simulink model "ultra"  (R2020b)
settings: Solver=FixedStepDiscrete  StartTime=0.0  StopTime=10.0  FixedStep=0.0005  RelTol=1e-3  EnableMultiTasking=on
undefined symbols (not defined in the file): acc_calmax1, acc_calmax2, acc_calmin1, acc_calmin2, akemancanshu, bre, bre_calmax, bre_calmin, ecucoder_acal, I_AN01_5K1, I_AN03_5V, I_AN04_5V, kd, ki, kp, leftmax, O_SW06_HS1A, rightmax, T_add, T_del, tiaoshi, zhiling
libraries: ec5744lib x215, canmsglib x75, simulink x10
(part 1 of 7)
settings Model: Creator=Tom liu  LastModifiedBy=Liu keliang
settings OptimizationCC: DefaultParameterBehavior=Inlined  UseDivisionForNetSlopeComputation=on  GainParamInheritBuiltInType=on  UseFloatMulNetSlope=on  InlineInvariantSignals=on  EnhancedBackFolding=on  ExpressionFolding=off  PassReuseOutputArgsAs=Individual arguments  RollThreshold=65  StateBitsets=on  DataBitsets=on  ZeroExternalMemoryAtStartup=off  ZeroInternalMemoryAtStartup=off  NoFixptDivByZeroProtection=on  EfficientFloat2IntCast=on  OptimizeBlockOrder=speed  DifferentSizesBufferReuse=on  EfficientTunableParamExpr=on
settings DebuggingCC: InheritedTsInSrcMsg=none  MultiTaskDSMMsg=none  ParameterTunabilityLossMsg=error
settings HardwareCC: ProdBitPerPointer=32  ProdBitPerSizeT=32  ProdBitPerPtrDiffT=32  ProdLargestAtomicInteger=Long  ProdLargestAtomicFloat=Double  ProdEndianess=BigEndian  ProdWordSize=32  ProdHWDeviceType=Freescale MPC5500  TargetBitPerPointer=64  TargetBitPerSizeT=64  TargetBitPerPtrDiffT=64  TargetLongLongMode=on  TargetIntDivRoundTo=Zero  TargetEndianess=LittleEndian  TargetWordSize=64  TargetHWDeviceType=MATLAB Host  ProdEqTarget=off
settings SFSimCC: MATLABDynamicMemAlloc=off  CustomCodeUndefinedFunction=UseInterfaceOnly
settings RTWCC: Description=Target for EC5744  SystemTargetFile=ec5744.tlc  MakeCommand=make_rtw optimized_fixed_point=1  GenerateMakefile=off  TemplateMakefile=ec5744_lcc.tmf  PostCodeGenCommand=ec5744_pst_s2(buildInfo)  GenerateReport=on  IncludeHyperlinkInReport=on  LaunchReport=on
settings CodeAppCC: ForceParamTrailComments=on  IgnoreCustomStorageClasses=off  OperatorAnnotations=on  SimulinkDataObjDesc=on  SFDataObjDesc=on  CustomSymbolStrGlobalVar=rt$N$M  CustomSymbolStrType=$N$M  CustomSymbolStrFcn=$N$M$F  CustomSymbolStrMacro=$N$M  InsertBlockDesc=on
settings STFCustomTargetCC: TargetLangStandard=C99 (ISO)  MultiwordLength=256  ModelReferenceCompliant=off  ConcurrentExecutionCompliant=off  IncludeMdlTerminateFcn=off  CombineOutputUpdateFcns=on  SuppressErrorStatus=on  ERTCustomFileBanners=on  SupportContinuousTime=off  SupportNonInlinedSFcns=off  RemoveResetFunc=on  MATLABClassNameForMDSCustomization=Simulink.SoftwareTarget.ERTCustomization  CPPClassGenCompliant=off  GRTInterface=off  SystemTargetFile=ec5744.tlc
settings ERTTargetCC: TargetLangStandard=C99 (ISO)  ModelReferenceCompliant=off  ParMdlRefBuildCompliant=off  CompOptLevelCompliant=off  ConcurrentExecutionCompliant=off  IncludeMdlTerminateFcn=off  SuppressErrorStatus=on  ModelStepFunctionPrototypeControlCompliant=off  CPPClassGenCompliant=off  UseToolchainInfoCompliant=off  GenerateASAP2=on  InlinedParameterPlacement=NonHierarchical  ERTSrcFileBannerTemplate=ec5744_code_template.cgt  ERTHdrFileBannerTemplate=ec5744_code_template.cgt  ERTDataSrcFileTemplate=ec5744_code_template.cgt  ERTDataHdrFileTemplate=ec5744_code_template.cgt  ERTCustomFileTemplate=ec5744_file_process.tlc

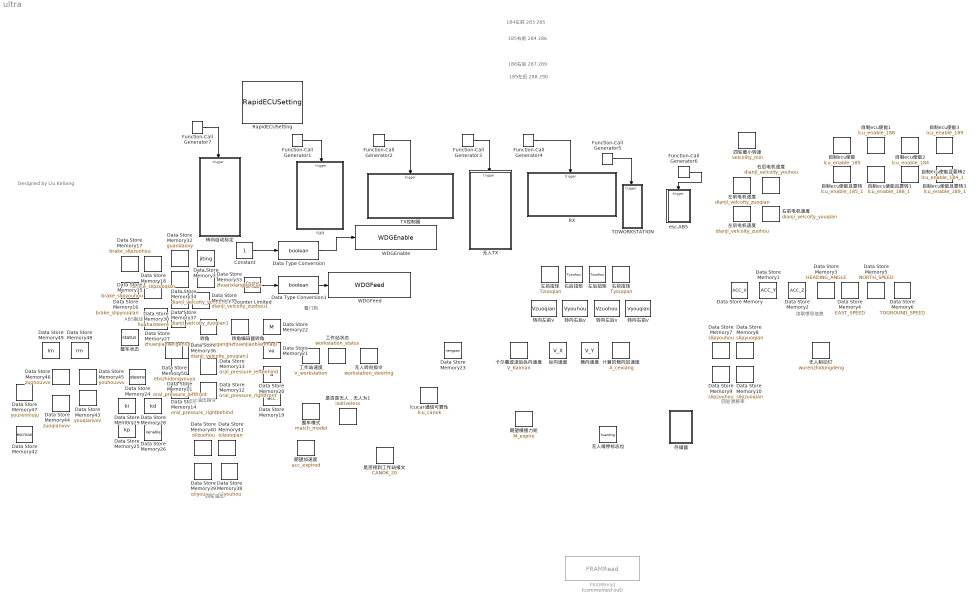
== system ultra ==
  note: Designed by Liu Keliang
  note: 四轮油压
  note: ABS制动
  note: esc油压指令
  note: 四轮滑移率
  note: 读取惯导信息
  note: 看门狗
  note: 189左后 288 290
  note: 188右后 287 289
  note: 185右前 284 286
  note: 184左前 283 285
  Constant : Constant
  Counter Limited : simulink/Sources/Counter Limited  uplimit=1  tsamp=0.01
  Data Store Memory : DataStoreMemory  DataStoreName=ACC_X  ReadBeforeWriteMsg=warning  WriteAfterWriteMsg=warning  WriteAfterReadMsg=warning  ShowAdditionalParam=off
  Data Store Memory1 : DataStoreMemory  DataStoreName=ACC_Y  ReadBeforeWriteMsg=warning  WriteAfterWriteMsg=warning  WriteAfterReadMsg=warning  ShowAdditionalParam=off
  Data Store Memory10 : DataStoreMemory  DataStoreName=slipzuoqian  ReadBeforeWriteMsg=warning  WriteAfterWriteMsg=warning  WriteAfterReadMsg=warning  ShowAdditionalParam=off
  Data Store Memory11 : DataStoreMemory  DataStoreName=oral_pressure_leftfront  ReadBeforeWriteMsg=warning  WriteAfterWriteMsg=warning  WriteAfterReadMsg=warning  ShowAdditionalParam=off
  Data Store Memory12 : DataStoreMemory  DataStoreName=oral_pressure_rightfront  ReadBeforeWriteMsg=warning  WriteAfterWriteMsg=warning  WriteAfterReadMsg=warning  ShowAdditionalParam=off
  Data Store Memory13 : DataStoreMemory  DataStoreName=oral_pressure_leftbehind  ReadBeforeWriteMsg=warning  WriteAfterWriteMsg=warning  WriteAfterReadMsg=warning  ShowAdditionalParam=off
  Data Store Memory14 : DataStoreMemory  DataStoreName=oral_pressure_rightbehind  ReadBeforeWriteMsg=warning  WriteAfterWriteMsg=warning  WriteAfterReadMsg=warning  ShowAdditionalParam=off
  Data Store Memory15 : DataStoreMemory  DataStoreName=brake_slipyouhou  ReadBeforeWriteMsg=warning  WriteAfterWriteMsg=warning  WriteAfterReadMsg=warning  ShowAdditionalParam=off
  Data Store Memory16 : DataStoreMemory  DataStoreName=brake_slipyouqian  ReadBeforeWriteMsg=warning  WriteAfterWriteMsg=warning  WriteAfterReadMsg=warning  ShowAdditionalParam=off
  Data Store Memory17 : DataStoreMemory  DataStoreName=brake_slipzuohou  ReadBeforeWriteMsg=warning  WriteAfterWriteMsg=warning  WriteAfterReadMsg=warning  ShowAdditionalParam=off
  Data Store Memory18 : DataStoreMemory  DataStoreName=brake_slipzuoqian  ReadBeforeWriteMsg=warning  WriteAfterWriteMsg=warning  WriteAfterReadMsg=warning  ShowAdditionalParam=off
  Data Store Memory19 : DataStoreMemory  DataStoreName=acc  ReadBeforeWriteMsg=warning  WriteAfterWriteMsg=warning  WriteAfterReadMsg=warning  ShowAdditionalParam=off
  Data Store Memory2 : DataStoreMemory  DataStoreName=ACC_Z  ReadBeforeWriteMsg=warning  WriteAfterWriteMsg=warning  WriteAfterReadMsg=warning  ShowAdditionalParam=off
  Data Store Memory20 : DataStoreMemory  DataStoreName=a  ReadBeforeWriteMsg=warning  WriteAfterWriteMsg=warning  WriteAfterReadMsg=warning  ShowAdditionalParam=off
  Data Store Memory21 : DataStoreMemory  DataStoreName=ve  ReadBeforeWriteMsg=warning  WriteAfterWriteMsg=warning  WriteAfterReadMsg=warning  ShowAdditionalParam=off
  Data Store Memory22 : DataStoreMemory  DataStoreName=M  ReadBeforeWriteMsg=warning  WriteAfterWriteMsg=warning  WriteAfterReadMsg=warning  ShowAdditionalParam=off
  Data Store Memory23 : DataStoreMemory  DataStoreName=nengpao  ReadBeforeWriteMsg=warning  WriteAfterWriteMsg=warning  WriteAfterReadMsg=warning  ShowAdditionalParam=off
  Data Store Memory24 : DataStoreMemory  DataStoreName=steere  ReadBeforeWriteMsg=warning  WriteAfterWriteMsg=warning  WriteAfterReadMsg=warning  ShowAdditionalParam=off
  Data Store Memory25 : DataStoreMemory  DataStoreName=kp  ReadBeforeWriteMsg=warning  WriteAfterWriteMsg=warning  WriteAfterReadMsg=warning  ShowAdditionalParam=off
  Data Store Memory26 : DataStoreMemory  DataStoreName=kenable  ReadBeforeWriteMsg=warning  WriteAfterWriteMsg=warning  WriteAfterReadMsg=warning  ShowAdditionalParam=off
  Data Store Memory27 : DataStoreMemory  DataStoreName=zhuanjiaoweigeniubi  ReadBeforeWriteMsg=warning  WriteAfterWriteMsg=warning  WriteAfterReadMsg=warning  ShowAdditionalParam=off
  Data Store Memory28 : DataStoreMemory  DataStoreName=kd  ReadBeforeWriteMsg=warning  WriteAfterWriteMsg=warning  WriteAfterReadMsg=warning  ShowAdditionalParam=off
  Data Store Memory29 : DataStoreMemory  DataStoreName=ki  ReadBeforeWriteMsg=warning  WriteAfterWriteMsg=warning  WriteAfterReadMsg=warning  ShowAdditionalParam=off
  Data Store Memory3 : DataStoreMemory  DataStoreName=HEADING_ANGLE  ReadBeforeWriteMsg=warning  WriteAfterWriteMsg=warning  WriteAfterReadMsg=warning  ShowAdditionalParam=off
  Data Store Memory30 : DataStoreMemory  DataStoreName=huahaisteere  ReadBeforeWriteMsg=warning  WriteAfterWriteMsg=warning  WriteAfterReadMsg=warning  ShowAdditionalParam=off
  Data Store Memory31 : DataStoreMemory  DataStoreName=jiting  ReadBeforeWriteMsg=warning  WriteAfterWriteMsg=warning  WriteAfterReadMsg=warning  ShowAdditionalParam=off
  Data Store Memory32 : DataStoreMemory  DataStoreName=guandaovy  ReadBeforeWriteMsg=warning  WriteAfterWriteMsg=warning  WriteAfterReadMsg=warning  ShowAdditionalParam=off
  Data Store Memory33 : DataStoreMemory  DataStoreName=zhuanxiangbaocuo  ReadBeforeWriteMsg=warning  WriteAfterWriteMsg=warning  WriteAfterReadMsg=warning  ShowAdditionalParam=off
  Data Store Memory34 : DataStoreMemory  DataStoreName=dianji_velcoity_youhou1  ReadBeforeWriteMsg=warning  WriteAfterWriteMsg=warning  WriteAfterReadMsg=warning  ShowAdditionalParam=off
  Data Store Memory35 : DataStoreMemory  DataStoreName=dianji_velcoity_zuohou1  ReadBeforeWriteMsg=warning  WriteAfterWriteMsg=warning  WriteAfterReadMsg=warning  ShowAdditionalParam=off
  Data Store Memory36 : DataStoreMemory  DataStoreName=dianji_velcoity_youqian1  ReadBeforeWriteMsg=warning  WriteAfterWriteMsg=warning  WriteAfterReadMsg=warning  ShowAdditionalParam=off
  Data Store Memory37 : DataStoreMemory  DataStoreName=dianji_velcoity_zuoqian1  ReadBeforeWriteMsg=warning  WriteAfterWriteMsg=warning  WriteAfterReadMsg=warning  ShowAdditionalParam=off
  Data Store Memory38 : DataStoreMemory  DataStoreName=oilyouhou  ReadBeforeWriteMsg=warning  WriteAfterWriteMsg=warning  WriteAfterReadMsg=warning  ShowAdditionalParam=off
  Data Store Memory39 : DataStoreMemory  DataStoreName=oilyouqian  ReadBeforeWriteMsg=warning  WriteAfterWriteMsg=warning  WriteAfterReadMsg=warning  ShowAdditionalParam=off
  Data Store Memory4 : DataStoreMemory  DataStoreName=EAST_SPEED  ReadBeforeWriteMsg=warning  WriteAfterWriteMsg=warning  WriteAfterReadMsg=warning  ShowAdditionalParam=off
  Data Store Memory40 : DataStoreMemory  DataStoreName=oilzuohou  ReadBeforeWriteMsg=warning  WriteAfterWriteMsg=warning  WriteAfterReadMsg=warning  ShowAdditionalParam=off
  Data Store Memory41 : DataStoreMemory  DataStoreName=oilzuoqian  ReadBeforeWriteMsg=warning  WriteAfterWriteMsg=warning  WriteAfterReadMsg=warning  ShowAdditionalParam=off
  Data Store Memory42 : DataStoreMemory  DataStoreName=escmax  ReadBeforeWriteMsg=warning  WriteAfterWriteMsg=warning  WriteAfterReadMsg=warning  ShowAdditionalParam=off
  Data Store Memory43 : DataStoreMemory  DataStoreName=youqianvvv  ReadBeforeWriteMsg=warning  WriteAfterWriteMsg=warning  WriteAfterReadMsg=warning  ShowAdditionalParam=off
  Data Store Memory44 : DataStoreMemory  DataStoreName=zuoqianvvv  ReadBeforeWriteMsg=warning  WriteAfterWriteMsg=warning  WriteAfterReadMsg=warning  ShowAdditionalParam=off
  Data Store Memory45 : DataStoreMemory  DataStoreName=youhouvvv  ReadBeforeWriteMsg=warning  WriteAfterWriteMsg=warning  WriteAfterReadMsg=warning  ShowAdditionalParam=off
  Data Store Memory46 : DataStoreMemory  DataStoreName=zuohouvvv  ReadBeforeWriteMsg=warning  WriteAfterWriteMsg=warning  WriteAfterReadMsg=warning  ShowAdditionalParam=off
  Data Store Memory47 : DataStoreMemory  DataStoreName=yourenniuju  ReadBeforeWriteMsg=warning  WriteAfterWriteMsg=warning  WriteAfterReadMsg=warning  ShowAdditionalParam=off
  Data Store Memory48 : DataStoreMemory  DataStoreName=rm  ReadBeforeWriteMsg=warning  WriteAfterWriteMsg=warning  WriteAfterReadMsg=warning  ShowAdditionalParam=off
  Data Store Memory49 : DataStoreMemory  DataStoreName=lm  ReadBeforeWriteMsg=warning  WriteAfterWriteMsg=warning  WriteAfterReadMsg=warning  ShowAdditionalParam=off
  Data Store Memory5 : DataStoreMemory  DataStoreName=NORTH_SPEED  ReadBeforeWriteMsg=warning  WriteAfterWriteMsg=warning  WriteAfterReadMsg=warning  ShowAdditionalParam=off
  Data Store Memory50 : DataStoreMemory  DataStoreName=ebszhidongyouya  ReadBeforeWriteMsg=warning  WriteAfterWriteMsg=warning  WriteAfterReadMsg=warning  ShowAdditionalParam=off
  Data Store Memory6 : DataStoreMemory  DataStoreName=TOGROUND_SPEED  ReadBeforeWriteMsg=warning  WriteAfterWriteMsg=warning  WriteAfterReadMsg=warning  ShowAdditionalParam=off
  Data Store Memory7 : DataStoreMemory  DataStoreName=slipyouhou  ReadBeforeWriteMsg=warning  WriteAfterWriteMsg=warning  WriteAfterReadMsg=warning  ShowAdditionalParam=off
  Data Store Memory8 : DataStoreMemory  DataStoreName=slipyuoqian  ReadBeforeWriteMsg=warning  WriteAfterWriteMsg=warning  WriteAfterReadMsg=warning  ShowAdditionalParam=off
  Data Store Memory9 : DataStoreMemory  DataStoreName=slipzuohou  ReadBeforeWriteMsg=warning  WriteAfterWriteMsg=warning  WriteAfterReadMsg=warning  ShowAdditionalParam=off
  Data Type Conversion : DataTypeConversion  OutDataTypeStr=boolean
  Data Type Conversion1 : DataTypeConversion  OutDataTypeStr=boolean
  FRAMRead : ec5744lib/RapidECU_U4B/12EEModule/FRAMRead  Commented=on  buffer=0  sampletime=-1
      settings: SourceProductName=ECUCoder for MPC5744
  Function-Call Generator1 : simulink/Ports & Subsystems/Function-Call Generator  sample_time=0.02  numberOfIterations=1  DisallowWideOutput=off
  Function-Call Generator2 : simulink/Ports & Subsystems/Function-Call Generator  sample_time=0.01  numberOfIterations=1  DisallowWideOutput=off
  Function-Call Generator3 : simulink/Ports & Subsystems/Function-Call Generator  sample_time=0.01  numberOfIterations=1  DisallowWideOutput=off
  Function-Call Generator4 : simulink/Ports & Subsystems/Function-Call Generator  sample_time=0.02  numberOfIterations=1  DisallowWideOutput=off
  Function-Call Generator5 : simulink/Ports & Subsystems/Function-Call Generator  sample_time=0.02  numberOfIterations=1  DisallowWideOutput=off
  Function-Call Generator6 : simulink/Ports & Subsystems/Function-Call Generator  sample_time=0.1  numberOfIterations=1  DisallowWideOutput=off
  Function-Call Generator7 : simulink/Ports & Subsystems/Function-Call Generator  sample_time=1  numberOfIterations=1  DisallowWideOutput=off
  RX : Subsystem  TreatAsAtomicUnit=on
  RapidECUSetting : ec5744lib/RapidECU_U4B/RapidECUSetting
      link override CAN: apdf=4  bpdf=4  cpdf=4
      link override LIN: abrt=19200
      settings: SourceProductName=ECUCoder for MPC5744
  TOWORKSTATION : Subsystem
  TX控制器 : Subsystem  TreatAsAtomicUnit=on
  WDGEnable : ec5744lib/RapidECU_U4B/08MCUManagement/WDGEnable  sampletime=-1
      settings: SourceProductName=ECUCoder for MPC5744
  WDGFeed : ec5744lib/RapidECU_U4B/08MCUManagement/WDGFeed  sampletime=-1
      settings: SourceProductName=ECUCoder for MPC5744
  esc,ABS : Subsystem
  lcucan通信可靠性 : DataStoreMemory  DataStoreName=lcu_canok  ReadBeforeWriteMsg=warning  WriteAfterWriteMsg=warning  WriteAfterReadMsg=warning  ShowAdditionalParam=off
  run : Subsystem
  卡尔曼滤波后纵向速度 : DataStoreMemory  DataStoreName=V_Kalman  ReadBeforeWriteMsg=warning  WriteAfterWriteMsg=warning  WriteAfterReadMsg=warning  ShowAdditionalParam=off
  右前扭矩 : DataStoreMemory  DataStoreName=Tyouqian  ReadBeforeWriteMsg=warning  WriteAfterWriteMsg=warning  WriteAfterReadMsg=warning  ShowAdditionalParam=off
  右前电机速度 : DataStoreMemory  DataStoreName=dianji_velcoity_youqian  ReadBeforeWriteMsg=warning  WriteAfterWriteMsg=warning  WriteAfterReadMsg=warning  ShowAdditionalParam=off
  右后扭矩 : DataStoreMemory  DataStoreName=Tyouhou  ReadBeforeWriteMsg=warning  WriteAfterWriteMsg=warning  WriteAfterReadMsg=warning  ShowAdditionalParam=off
  右后电机速度 : DataStoreMemory  DataStoreName=dianji_velcoity_youhou  ReadBeforeWriteMsg=warning  WriteAfterWriteMsg=warning  WriteAfterReadMsg=warning  ShowAdditionalParam=off
  四轮最小转速 : DataStoreMemory  DataStoreName=velcolity_min  ReadBeforeWriteMsg=warning  WriteAfterWriteMsg=warning  WriteAfterReadMsg=warning  ShowAdditionalParam=off
  存储器 : Subsystem
  工作站状态 : DataStoreMemory  DataStoreName=workstation_status  ReadBeforeWriteMsg=warning  WriteAfterWriteMsg=warning  WriteAfterReadMsg=warning  ShowAdditionalParam=off
  工作站速度 : DataStoreMemory  DataStoreName=V_workstation  ReadBeforeWriteMsg=warning  WriteAfterWriteMsg=warning  WriteAfterReadMsg=warning  ShowAdditionalParam=off
  左前扭矩 : DataStoreMemory  DataStoreName=Tzuoqian  ReadBeforeWriteMsg=warning  WriteAfterWriteMsg=warning  WriteAfterReadMsg=warning  ShowAdditionalParam=off
  左前电机速度 : DataStoreMemory  DataStoreName=dianji_velcoity_zuoqian  ReadBeforeWriteMsg=warning  WriteAfterWriteMsg=warning  WriteAfterReadMsg=warning  ShowAdditionalParam=off
  左后扭矩 : DataStoreMemory  DataStoreName=Tzuohou  ReadBeforeWriteMsg=warning  WriteAfterWriteMsg=warning  WriteAfterReadMsg=warning  ShowAdditionalParam=off
  左后电机速度 : DataStoreMemory  DataStoreName=dianji_velcoity_zuohou  ReadBeforeWriteMsg=warning  WriteAfterWriteMsg=warning  WriteAfterReadMsg=warning  ShowAdditionalParam=off
  整车模式 : DataStoreMemory  DataStoreName=match_model  ReadBeforeWriteMsg=warning  WriteAfterWriteMsg=warning  WriteAfterReadMsg=warning  ShowAdditionalParam=off
  整车状态 : DataStoreMemory  DataStoreName=status  ReadBeforeWriteMsg=warning  WriteAfterWriteMsg=warning  WriteAfterReadMsg=warning  ShowAdditionalParam=off
  无人TX : Subsystem
  无人制动灯 : DataStoreMemory  DataStoreName=wurenzhidongdeng  ReadBeforeWriteMsg=warning  WriteAfterWriteMsg=warning  WriteAfterReadMsg=warning  ShowAdditionalParam=off
  无人缓停标志位 : DataStoreMemory  DataStoreName=huanting  ReadBeforeWriteMsg=warning  WriteAfterWriteMsg=warning  WriteAfterReadMsg=warning  ShowAdditionalParam=off
  无人转向指令 : DataStoreMemory  DataStoreName=workstation_steering  ReadBeforeWriteMsg=warning  WriteAfterWriteMsg=warning  WriteAfterReadMsg=warning  ShowAdditionalParam=off
  是否接到工作站报文 : DataStoreMemory  DataStoreName=CANOK_20  ReadBeforeWriteMsg=warning  WriteAfterWriteMsg=warning  WriteAfterReadMsg=warning  ShowAdditionalParam=off
  是否是无人，无人为1 : DataStoreMemory  DataStoreName=isdriveless  ReadBeforeWriteMsg=warning  WriteAfterWriteMsg=warning  WriteAfterReadMsg=warning  ShowAdditionalParam=off
  期望加速度 : DataStoreMemory  DataStoreName=acc_expired  ReadBeforeWriteMsg=warning  WriteAfterWriteMsg=warning  WriteAfterReadMsg=warning  ShowAdditionalParam=off
  期望横摆力矩 : DataStoreMemory  DataStoreName=M_expire  ReadBeforeWriteMsg=warning  WriteAfterWriteMsg=warning  WriteAfterReadMsg=warning  ShowAdditionalParam=off
  横向速度 : DataStoreMemory  DataStoreName=V_Y  ReadBeforeWriteMsg=warning  WriteAfterWriteMsg=warning  WriteAfterReadMsg=warning  ShowAdditionalParam=off
  纵向速度 : DataStoreMemory  DataStoreName=V_X  ReadBeforeWriteMsg=warning  WriteAfterWriteMsg=warning  WriteAfterReadMsg=warning  ShowAdditionalParam=off
  自制ecu使能 : DataStoreMemory  DataStoreName=lcu_enable_185  ReadBeforeWriteMsg=warning  WriteAfterWriteMsg=warning  WriteAfterReadMsg=warning  ShowAdditionalParam=off
  自制ecu使能1 : DataStoreMemory  DataStoreName=lcu_enable_188  ReadBeforeWriteMsg=warning  WriteAfterWriteMsg=warning  WriteAfterReadMsg=warning  ShowAdditionalParam=off
  自制ecu使能2 : DataStoreMemory  DataStoreName=lcu_enable_184  ReadBeforeWriteMsg=warning  WriteAfterWriteMsg=warning  WriteAfterReadMsg=warning  ShowAdditionalParam=off
  自制ecu使能3 : DataStoreMemory  DataStoreName=lcu_enable_189  ReadBeforeWriteMsg=warning  WriteAfterWriteMsg=warning  WriteAfterReadMsg=warning  ShowAdditionalParam=off
  自制ecu使能且要转 : DataStoreMemory  DataStoreName=lcu_enable_185_1  ReadBeforeWriteMsg=warning  WriteAfterWriteMsg=warning  WriteAfterReadMsg=warning  ShowAdditionalParam=off
  自制ecu使能且要转1 : DataStoreMemory  DataStoreName=lcu_enable_188_1  ReadBeforeWriteMsg=warning  WriteAfterWriteMsg=warning  WriteAfterReadMsg=warning  ShowAdditionalParam=off
  自制ecu使能且要转2 : DataStoreMemory  DataStoreName=lcu_enable_184_1  ReadBeforeWriteMsg=warning  WriteAfterWriteMsg=warning  WriteAfterReadMsg=warning  ShowAdditionalParam=off
  自制ecu使能且要转3 : DataStoreMemory  DataStoreName=lcu_enable_189_1  ReadBeforeWriteMsg=warning  WriteAfterWriteMsg=warning  WriteAfterReadMsg=warning  ShowAdditionalParam=off
  计算的侧向加速度 : DataStoreMemory  DataStoreName=A_cexiang  ReadBeforeWriteMsg=warning  WriteAfterWriteMsg=warning  WriteAfterReadMsg=warning  ShowAdditionalParam=off
  转向右前v : DataStoreMemory  DataStoreName=Vyouqian  ReadBeforeWriteMsg=warning  WriteAfterWriteMsg=warning  WriteAfterReadMsg=warning  ShowAdditionalParam=off
  转向右后v : DataStoreMemory  DataStoreName=Vyouhou  ReadBeforeWriteMsg=warning  WriteAfterWriteMsg=warning  WriteAfterReadMsg=warning  ShowAdditionalParam=off
  转向左前v : DataStoreMemory  DataStoreName=Vzuoqian  ReadBeforeWriteMsg=warning  WriteAfterWriteMsg=warning  WriteAfterReadMsg=warning  ShowAdditionalParam=off
  转向左后v : DataStoreMemory  DataStoreName=Vzuohou  ReadBeforeWriteMsg=warning  WriteAfterWriteMsg=warning  WriteAfterReadMsg=warning  ShowAdditionalParam=off
  转向自动标定 : Subsystem
  转角 : DataStoreMemory  DataStoreName=steeringangle  ReadBeforeWriteMsg=warning  WriteAfterWriteMsg=warning  WriteAfterReadMsg=warning  ShowAdditionalParam=off
  转角编码器转角 : DataStoreMemory  DataStoreName=zhuanjiaobianmaqi  ReadBeforeWriteMsg=warning  WriteAfterWriteMsg=warning  WriteAfterReadMsg=warning  ShowAdditionalParam=off
  wires:
  Function-Call Generator4/1 -> RX/Trigger
  Function-Call Generator2/1 -> TX控制器/Trigger
  Function-Call Generator1/1 -> run/Trigger
  Constant/1 -> Data Type Conversion/1
  Data Type Conversion/1 -> WDGEnable/1
  Data Type Conversion1/1 -> WDGFeed/1
  Counter Limited/1 -> Data Type Conversion1/1
  Function-Call Generator3/1 -> 无人TX/Trigger
  Function-Call Generator5/1 -> TOWORKSTATION/Trigger
  Function-Call Generator6/1 -> esc,ABS/Trigger
  Function-Call Generator7/1 -> 转向自动标定/Trigger

== system ultra/RX ==
  function : TriggerPort  TriggerType=function-call  VariantControl=Variant
  283 285左前 : Subsystem
  284 286右前 : Subsystem
  287 289右后 : Subsystem
  288 290左后 : Subsystem
  ebs : Subsystem
  lcu——receive : Subsystem
  工作站 : Subsystem
  惯导 : Subsystem
  转向——receive1 : Subsystem
  转向——receive编码器 : Subsystem

== system ultra/TOWORKSTATION ==
  function : TriggerPort  TriggerType=function-call  VariantControl=Variant
  Data Store Read : DataStoreRead  DataStoreName=match_model
  MATLAB Function : MATLAB Function  TreatAsAtomicUnit=on
  toworkstation : Subsystem
  转向 : Subsystem
  wires:
  Data Store Read/1 -> MATLAB Function/1(u)
  MATLAB Function/1(y) -> toworkstation/Enable

== system ultra/TX控制器 ==
  function : TriggerPort  TriggerType=function-call  VariantControl=Variant
  CAN Pack : canmsglib/CAN Pack  Commented=on  CANdbFile=C:\Users\Liu keliang\Desktop\HRT2023\HRT23赛季刘科良\CANdbc\zhuanjiaobianmaqiceshiTX.dbc  MsgList=ceshi  MsgName=ceshi  MsgIDType=Standard (11-bit identifier)  MsgIdentifier=136  MsgLength=2  Remote=off  ApplyMinMax=off  BusOutput=off  SignalInfo={'New_Signal_1','0','16','LE','unsigned','Standard','0','1','0','-Inf','Inf'}
      settings: SourceProductBaseCode=ME,XP,VN  DataFormat=CANdb specified signals
  CAN Pack1 : canmsglib/CAN Pack  Commented=on  CANdbFile=C:\Users\Liu keliang\Desktop\HRT2023\HRT23赛季刘科良\CANdbc\version.dbc  MsgList=New_Message_2  MsgName=New_Message_2  MsgIDType=Standard (11-bit identifier)  MsgIdentifier=819  MsgLength=1  Remote=off  ApplyMinMax=off  BusOutput=off  SignalInfo={'New_Signal_9','0','8','LE','signed','Standard','0','1','0','-Inf','Inf'}
      settings: SourceProductBaseCode=ME,XP,VN  DataFormat=CANdb specified signals
  CANPackMessage : ec5744lib/RapidECU_U4B/04CANCommunication/CANPackMessage  Commented=on  datalength=2  sampletime=-1
      settings: SourceProductName=ECUCoder for MPC5744
  CANPackMessage1 : ec5744lib/RapidECU_U4B/04CANCommunication/CANPackMessage  Commented=on  datalength=1  sampletime=-1
      settings: SourceProductName=ECUCoder for MPC5744
  CANTransmit : ec5744lib/RapidECU_U4B/04CANCommunication/CANTransmit  Commented=on  canmodule=1  canbuffer=63  canmessageid=hex2dec('88')  canmessagetype=Standard(11-bit ID)  datalength=2  sampletime=-1
      settings: SourceProductName=ECUCoder for MPC5744
  CANTransmit1 : ec5744lib/RapidECU_U4B/04CANCommunication/CANTransmit  Commented=on  canmodule=0  canbuffer=12  canmessageid=hex2dec('333')  canmessagetype=Standard(11-bit ID)  datalength=1  sampletime=-1
      settings: SourceProductName=ECUCoder for MPC5744
  Constant : Constant  Commented=on  Value=2  SampleTime=-1
  Data Store Read : DataStoreRead  DataStoreName=V_workstation
  Data Store Read1 : DataStoreRead  Commented=on  DataStoreName=zhuanjiaobianmaqi
  Data Store Read2 : DataStoreRead  DataStoreName=match_model
  Data Store Read3 : DataStoreRead  DataStoreName=match_model
  Data Store Read5 : DataStoreRead  DataStoreName=V_workstation
  Data Store Read6 : DataStoreRead  DataStoreName=workstation_steering
  Data Store Read9 : DataStoreRead  DataStoreName=V_Kalman
  Data Store Write : DataStoreWrite  DataStoreName=youqianvvv
  Data Store Write1 : DataStoreWrite  DataStoreName=zuoqianvvv
  Data Store Write2 : DataStoreWrite  DataStoreName=youhouvvv
  Data Store Write3 : DataStoreWrite  DataStoreName=zuohouvvv
  Data Type Conversion : DataTypeConversion  Commented=on  OutDataTypeStr=uint8
  Data Type Conversion1 : DataTypeConversion  Commented=on  OutDataTypeStr=uint8
  MATLAB Function : MATLAB Function  TreatAsAtomicUnit=on
  MATLAB Function1 : MATLAB Function  TreatAsAtomicUnit=on
  MeaModule : ec5744lib/RapidECU_U4B/07Calibration/MeaModule  Commented=on  signal=bianmaqi88
      settings: SourceProductName=ECUCoder for MPC5744
  Subsystem : Subsystem
  Subsystem1 : Subsystem
  Terminator : Terminator  Commented=on
  Terminator1 : Terminator  Commented=on
  扭矩 : Subsystem
  速度 : Subsystem
  wires:
  Data Store Read/1 -> MATLAB Function/1(u)
  MATLAB Function/2(yniuju) -> 扭矩/Enable
  MATLAB Function/1(ysudu) -> 速度/Enable
  Data Store Read2/1 -> MATLAB Function/2(model)
  Data Store Read9/1 -> MATLAB Function/3(v)
  CANTransmit/1 -> MeaModule/1
  Data Type Conversion/1 -> CANTransmit/1
  CANPackMessage/1 -> Data Type Conversion/1
  MeaModule/1 -> Terminator/1
  CAN Pack/1 -> CANPackMessage/1
  Data Store Read1/1 -> CAN Pack/1
  Data Store Read3/1 -> MATLAB Function1/1(model)
  MATLAB Function1/1(y) -> Subsystem/Enable
  Data Type Conversion1/1 -> CANTransmit1/1
  CAN Pack1/1 -> CANPackMessage1/1
  Constant/1 -> CAN Pack1/1
  CANTransmit1/1 -> Terminator1/1
  CANPackMessage1/1 -> Data Type Conversion1/1
  Data Store Read5/1 -> Subsystem1/2(v)
  Data Store Read6/1 -> Subsystem1/1(angle)
  Subsystem1/1(youqianvvv) -> Data Store Write/1
  Subsystem1/2(zuoqianvvv) -> Data Store Write1/1
  Subsystem1/3(youhouvvv) -> Data Store Write2/1
  Subsystem1/4(zuohouvvv) -> Data Store Write3/1

== system ultra/esc,ABS ==
  function : TriggerPort  TriggerType=function-call  VariantControl=Variant
  Data Store Read : DataStoreRead  DataStoreName=match_model
  MATLAB Function : MATLAB Function  TreatAsAtomicUnit=on
  Subsystem : Subsystem
  wires:
  Data Store Read/1 -> MATLAB Function/1(u)
  MATLAB Function/1(y) -> Subsystem/Enable

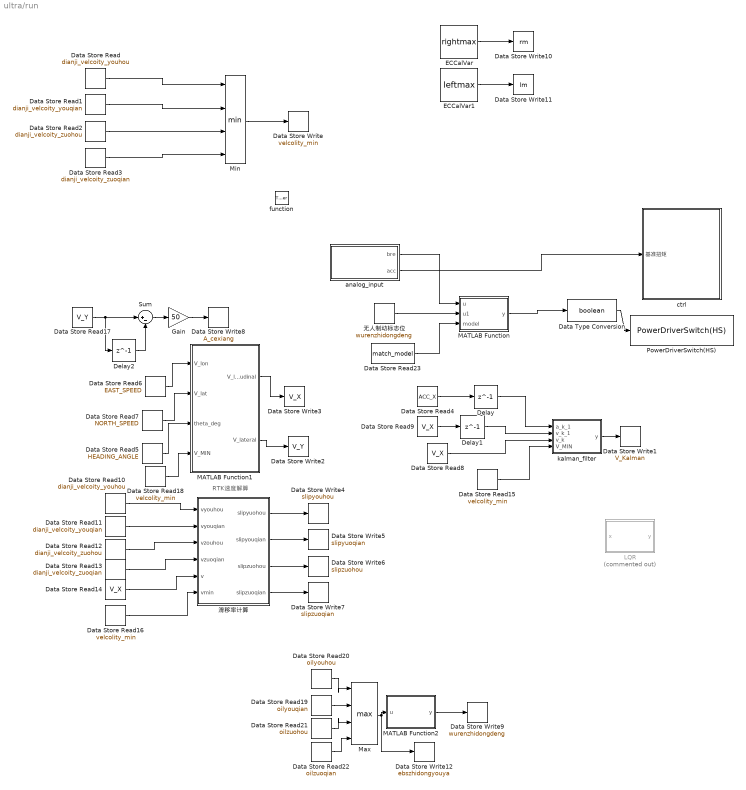
== system ultra/run ==
  note: RTK速度解算
  function : TriggerPort  TriggerType=function-call  VariantControl=Variant
  Data Store Read : DataStoreRead  DataStoreName=dianji_velcoity_youhou
  Data Store Read1 : DataStoreRead  DataStoreName=dianji_velcoity_youqian
  Data Store Read10 : DataStoreRead  DataStoreName=dianji_velcoity_youhou
  Data Store Read11 : DataStoreRead  DataStoreName=dianji_velcoity_youqian
  Data Store Read12 : DataStoreRead  DataStoreName=dianji_velcoity_zuohou
  Data Store Read13 : DataStoreRead  DataStoreName=dianji_velcoity_zuoqian
  Data Store Read14 : DataStoreRead  DataStoreName=V_X
  Data Store Read15 : DataStoreRead  DataStoreName=velcolity_min
  Data Store Read16 : DataStoreRead  DataStoreName=velcolity_min
  Data Store Read17 : DataStoreRead  DataStoreName=V_Y
  Data Store Read18 : DataStoreRead  DataStoreName=velcolity_min
  Data Store Read19 : DataStoreRead  DataStoreName=oilyouqian
  Data Store Read2 : DataStoreRead  DataStoreName=dianji_velcoity_zuohou
  Data Store Read20 : DataStoreRead  DataStoreName=oilyouhou
  Data Store Read21 : DataStoreRead  DataStoreName=oilzuohou
  Data Store Read22 : DataStoreRead  DataStoreName=oilzuoqian
  Data Store Read23 : DataStoreRead  DataStoreName=match_model
  Data Store Read3 : DataStoreRead  DataStoreName=dianji_velcoity_zuoqian
  Data Store Read4 : DataStoreRead  DataStoreName=ACC_X
  Data Store Read5 : DataStoreRead  DataStoreName=HEADING_ANGLE
  Data Store Read6 : DataStoreRead  DataStoreName=EAST_SPEED
  Data Store Read7 : DataStoreRead  DataStoreName=NORTH_SPEED
  Data Store Read8 : DataStoreRead  DataStoreName=V_X
  Data Store Read9 : DataStoreRead  DataStoreName=V_X
  Data Store Write : DataStoreWrite  DataStoreName=velcolity_min
  Data Store Write1 : DataStoreWrite  DataStoreName=V_Kalman
  Data Store Write10 : DataStoreWrite  DataStoreName=rm
  Data Store Write11 : DataStoreWrite  DataStoreName=lm
  Data Store Write12 : DataStoreWrite  DataStoreName=ebszhidongyouya
  Data Store Write2 : DataStoreWrite  DataStoreName=V_Y
  Data Store Write3 : DataStoreWrite  DataStoreName=V_X
  Data Store Write4 : DataStoreWrite  DataStoreName=slipyouhou
  Data Store Write5 : DataStoreWrite  DataStoreName=slipyuoqian
  Data Store Write6 : DataStoreWrite  DataStoreName=slipzuohou
  Data Store Write7 : DataStoreWrite  DataStoreName=slipzuoqian
  Data Store Write8 : DataStoreWrite  DataStoreName=A_cexiang
  Data Store Write9 : DataStoreWrite  DataStoreName=wurenzhidongdeng
  Data Type Conversion : DataTypeConversion  OutDataTypeStr=boolean
  Delay : Delay  DelayLength=1
  Delay1 : Delay  DelayLength=1
  Delay2 : Delay  DelayLength=1
  ECCalVar : Constant  InitFcn=ecucoder_acal;  Value=rightmax  OutDataTypeStr=Inherit: Inherit via back propagation  SampleTime=-1
  ECCalVar1 : Constant  InitFcn=ecucoder_acal;  Value=leftmax  OutDataTypeStr=Inherit: Inherit via back propagation  SampleTime=-1
  Gain : Gain  Gain=50
  LQR : MATLAB Function  Commented=on  TreatAsAtomicUnit=on
  MATLAB Function : MATLAB Function  TreatAsAtomicUnit=on
  MATLAB Function1 : MATLAB Function  TreatAsAtomicUnit=on
  MATLAB Function2 : MATLAB Function  TreatAsAtomicUnit=on
  Max : MinMax  Function=max  Inputs=4
  Min : MinMax  Inputs=4
  PowerDriverSwitch(HS) : ec5744lib/RapidECU_U4B/02PowerDriverSwitch/PowerDriverSwitch(HS)  channel=95:O_SW06_HS1A  sampletime=-1
      settings: SourceProductName=ECUCoder for MPC5744
  Sum : Sum  Inputs=|+-
  analog_input : Subsystem  TreatAsAtomicUnit=on
  ctrl : Subsystem
  kalman_filter : MATLAB Function  TreatAsAtomicUnit=on
  无人制动标志位 : DataStoreRead  DataStoreName=wurenzhidongdeng
  滑移率计算 : MATLAB Function  TreatAsAtomicUnit=on
  wires:
  Data Type Conversion/1 -> PowerDriverSwitch(HS)/1
  analog_input/2(acc) -> ctrl/1(基准扭矩)
  MATLAB Function/1(y) -> Data Type Conversion/1
  analog_input/1(bre) -> MATLAB Function/1(u)
  Min/1 -> Data Store Write/1
  kalman_filter/1(y) -> Data Store Write1/1
  Data Store Read5/1 -> MATLAB Function1/3(theta_deg)
  Data Store Read6/1 -> MATLAB Function1/1(V_lon)
  Data Store Read7/1 -> MATLAB Function1/2(V_lat)
  MATLAB Function1/2(V_lateral) -> Data Store Write2/1
  MATLAB Function1/1(V_longitudinal) -> Data Store Write3/1
  Data Store Read8/1 -> kalman_filter/3(v_k)
  Data Store Read4/1 -> Delay/1
  Delay/1 -> kalman_filter/1(a_k_1)
  Data Store Read9/1 -> Delay1/1
  Delay1/1 -> kalman_filter/2(v_k_1)
  Data Store Read13/1 -> 滑移率计算/4(vzuoqian)
  Data Store Read10/1 -> 滑移率计算/1(vyouhou)
  Data Store Read11/1 -> 滑移率计算/2(vyouqian)
  Data Store Read12/1 -> 滑移率计算/3(vzouhou)
  Data Store Read14/1 -> 滑移率计算/5(v)
  滑移率计算/1(slipyuohou) -> Data Store Write4/1
  滑移率计算/4(slipzuoqian) -> Data Store Write7/1
  滑移率计算/3(slipzuohou) -> Data Store Write6/1
  滑移率计算/2(slipyouqian) -> Data Store Write5/1
  Data Store Read15/1 -> kalman_filter/4(V_MIN)
  Data Store Read16/1 -> 滑移率计算/6(vmin)
  Data Store Read17/1 -> Delay2/1, Sum/1
  Delay2/1 -> Sum/2
  Sum/1 -> Gain/1
  Gain/1 -> Data Store Write8/1
  无人制动标志位/1 -> MATLAB Function/2(u1)
  Data Store Read18/1 -> MATLAB Function1/4(V_MIN)
  Data Store Read/1 -> Min/1
  Data Store Read1/1 -> Min/2
  Data Store Read2/1 -> Min/3
  Data Store Read3/1 -> Min/4
  Data Store Read20/1 -> Max/1
  Data Store Read19/1 -> Max/2
  Data Store Read21/1 -> Max/3
  Data Store Read22/1 -> Max/4
  Max/1 -> MATLAB Function2/1(u), Data Store Write12/1
  MATLAB Function2/1(y) -> Data Store Write9/1
  Data Store Read23/1 -> MATLAB Function/3(model)
  ECCalVar/1 -> Data Store Write10/1
  ECCalVar1/1 -> Data Store Write11/1

== system ultra/存储器 ==
  FRAMEnable1 : ec5744lib/RapidECU_U4B/12EEModule/FRAMEnable  framenable=on
      settings: SourceProductName=ECUCoder for MPC5744
  MeaModule : ec5744lib/RapidECU_U4B/07Calibration/MeaModule  signal=dddddddd
      settings: SourceProductName=ECUCoder for MPC5744
  MeaModule1 : ec5744lib/RapidECU_U4B/07Calibration/MeaModule  signal=kkkkkkkkkkk
      settings: SourceProductName=ECUCoder for MPC5744
  Terminator : Terminator
  Terminator1 : Terminator
  d : ec5744lib/RapidECU_U4B/12EEModule/FRAMRead  buffer=1  sampletime=-1
      settings: SourceProductName=ECUCoder for MPC5744
  k : ec5744lib/RapidECU_U4B/12EEModule/FRAMRead  buffer=0  sampletime=-1
      settings: SourceProductName=ECUCoder for MPC5744
  wires:
  k/1 -> MeaModule1/1
  d/1 -> MeaModule/1
  MeaModule1/1 -> Terminator/1
  MeaModule/1 -> Terminator1/1

== system ultra/无人TX ==
  function : TriggerPort  TriggerType=function-call  VariantControl=Variant
  Data Store Read1 : DataStoreRead  DataStoreName=match_model
  Data Store Read2 : DataStoreRead  DataStoreName=status
  Data Store Write : DataStoreWrite  DataStoreName=kp
  Data Store Write1 : DataStoreWrite  DataStoreName=ki
  Data Store Write2 : DataStoreWrite  DataStoreName=kd
  Data Store Write3 : DataStoreWrite  DataStoreName=kenable
  ECCalVar : Constant  InitFcn=ecucoder_acal;  Value=kp  OutDataTypeStr=Inherit: Inherit via back propagation  SampleTime=-1
  ECCalVar1 : Constant  InitFcn=ecucoder_acal;  Value=ki  OutDataTypeStr=Inherit: Inherit via back propagation  SampleTime=-1
  ECCalVar2 : Constant  InitFcn=ecucoder_acal;  Value=kd  OutDataTypeStr=Inherit: Inherit via back propagation  SampleTime=-1
  MATLAB Function1 : MATLAB Function  TreatAsAtomicUnit=on
  Max : MinMax  Inputs=3
  转向换算 : Subsystem
  wires:
  Data Store Read1/1 -> MATLAB Function1/1(model)
  MATLAB Function1/1(y) -> 转向换算/Enable
  Data Store Read2/1 -> MATLAB Function1/2(status)
  ECCalVar/1 -> Max/3, Data Store Write/1
  ECCalVar1/1 -> Max/2, Data Store Write1/1
  ECCalVar2/1 -> Max/1, Data Store Write2/1
  Max/1 -> Data Store Write3/1

== system ultra/转向自动标定 ==
  function : TriggerPort  TriggerType=function-call  VariantControl=Variant
  Data Store Read1 : DataStoreRead  DataStoreName=match_model
  Data Store Read2 : DataStoreRead  DataStoreName=status
  MATLAB Function1 : MATLAB Function  TreatAsAtomicUnit=on
  转向自动标定 : Subsystem
  wires:
  Data Store Read1/1 -> MATLAB Function1/1(model)
  MATLAB Function1/1(y) -> 转向自动标定/Enable
  Data Store Read2/1 -> MATLAB Function1/2(status)

== system ultra/RX/283 285左前 ==
  CANReceive1 : ec5744lib/RapidECU_U4B/04CANCommunication/CANReceive  canmodule=0  canbuffer=40  canmessageid=hex2dec('283')  canmessagetype=Standard(11-bit ID)  datalength=8  sampletime=-1
      settings: SourceProductName=ECUCoder for MPC5744
  CANReceive2 : ec5744lib/RapidECU_U4B/04CANCommunication/CANReceive  canmodule=0  canbuffer=41  canmessageid=hex2dec('285')  canmessagetype=Standard(11-bit ID)  datalength=8  sampletime=-1
      settings: SourceProductName=ECUCoder for MPC5744
  MeaModule1 : ec5744lib/RapidECU_U4B/07Calibration/MeaModule  signal=CANOK_283
      settings: SourceProductName=ECUCoder for MPC5744
  MeaModule2 : ec5744lib/RapidECU_U4B/07Calibration/MeaModule  signal=CANOK_285
      settings: SourceProductName=ECUCoder for MPC5744
  Subsystem1 : Subsystem
  Subsystem2 : Subsystem
  Terminator1 : Terminator
  Terminator3 : Terminator
  wires:
  CANReceive1/5 -> Terminator3/1
  CANReceive1/2 -> MeaModule1/1
  CANReceive1/1 -> Subsystem2/Trigger
  CANReceive1/3 -> Subsystem2/2(ID)
  CANReceive1/4 -> Subsystem2/3(msg)
  MeaModule1/1 -> Subsystem2/1(Enable)
  CANReceive2/3 -> Subsystem1/2(ID)
  CANReceive2/4 -> Subsystem1/3(msg)
  CANReceive2/5 -> Terminator1/1
  CANReceive2/1 -> Subsystem1/Trigger
  MeaModule2/1 -> Subsystem1/1(Enable)
  CANReceive2/2 -> MeaModule2/1

== system ultra/RX/284 286右前 ==
  CANReceive1 : ec5744lib/RapidECU_U4B/04CANCommunication/CANReceive  canmodule=0  canbuffer=42  canmessageid=hex2dec('284')  canmessagetype=Standard(11-bit ID)  datalength=8  sampletime=-1
      settings: SourceProductName=ECUCoder for MPC5744
  CANReceive2 : ec5744lib/RapidECU_U4B/04CANCommunication/CANReceive  canmodule=0  canbuffer=43  canmessageid=hex2dec('286')  canmessagetype=Standard(11-bit ID)  datalength=8  sampletime=-1
      settings: SourceProductName=ECUCoder for MPC5744
  MeaModule1 : ec5744lib/RapidECU_U4B/07Calibration/MeaModule  signal=CANOK_284
      settings: SourceProductName=ECUCoder for MPC5744
  MeaModule2 : ec5744lib/RapidECU_U4B/07Calibration/MeaModule  signal=CANOK_286
      settings: SourceProductName=ECUCoder for MPC5744
  Subsystem1 : Subsystem
  Subsystem2 : Subsystem
  Terminator1 : Terminator
  Terminator3 : Terminator
  wires:
  CANReceive1/5 -> Terminator3/1
  CANReceive1/2 -> MeaModule1/1
  CANReceive1/1 -> Subsystem2/Trigger
  CANReceive1/3 -> Subsystem2/2(ID)
  CANReceive1/4 -> Subsystem2/3(msg)
  MeaModule1/1 -> Subsystem2/1(Enable)
  CANReceive2/3 -> Subsystem1/2(ID)
  CANReceive2/4 -> Subsystem1/3(msg)
  CANReceive2/5 -> Terminator1/1
  CANReceive2/1 -> Subsystem1/Trigger
  MeaModule2/1 -> Subsystem1/1(Enable)
  CANReceive2/2 -> MeaModule2/1

== system ultra/RX/287 289右后 ==
  CANReceive1 : ec5744lib/RapidECU_U4B/04CANCommunication/CANReceive  Commented=on  canmodule=0  canbuffer=46  canmessageid=hex2dec('287')  canmessagetype=Standard(11-bit ID)  datalength=8  sampletime=-1
      settings: SourceProductName=ECUCoder for MPC5744
  CANReceive2 : ec5744lib/RapidECU_U4B/04CANCommunication/CANReceive  canmodule=0  canbuffer=47  canmessageid=hex2dec('289')  canmessagetype=Standard(11-bit ID)  datalength=8  sampletime=-1
      settings: SourceProductName=ECUCoder for MPC5744
  CANReceive3 : ec5744lib/RapidECU_U4B/04CANCommunication/CANReceive  canmodule=0  canbuffer=55  canmessageid=hex2dec('287')  canmessagetype=Standard(11-bit ID)  datalength=8  sampletime=-1
      settings: SourceProductName=ECUCoder for MPC5744
  MeaModule1 : ec5744lib/RapidECU_U4B/07Calibration/MeaModule  Commented=on  signal=CANOK_287
      settings: SourceProductName=ECUCoder for MPC5744
  MeaModule2 : ec5744lib/RapidECU_U4B/07Calibration/MeaModule  signal=CANOK_289
      settings: SourceProductName=ECUCoder for MPC5744
  MeaModule3 : ec5744lib/RapidECU_U4B/07Calibration/MeaModule  signal=CANOK_287
      settings: SourceProductName=ECUCoder for MPC5744
  Subsystem1 : Subsystem
  Subsystem2 : Subsystem  Commented=on
  Subsystem3 : Subsystem
  Terminator1 : Terminator
  Terminator2 : Terminator
  Terminator3 : Terminator  Commented=on
  wires:
  CANReceive1/5 -> Terminator3/1
  CANReceive1/2 -> MeaModule1/1
  CANReceive1/1 -> Subsystem2/Trigger
  CANReceive1/3 -> Subsystem2/2(ID)
  CANReceive1/4 -> Subsystem2/3(msg)
  MeaModule1/1 -> Subsystem2/1(Enable)
  CANReceive2/3 -> Subsystem1/2(ID)
  CANReceive2/4 -> Subsystem1/3(msg)
  CANReceive2/5 -> Terminator1/1
  CANReceive2/1 -> Subsystem1/Trigger
  MeaModule2/1 -> Subsystem1/1(Enable)
  CANReceive2/2 -> MeaModule2/1
  CANReceive3/2 -> MeaModule3/1
  CANReceive3/1 -> Subsystem3/Trigger
  CANReceive3/4 -> Subsystem3/3(msg)
  MeaModule3/1 -> Subsystem3/1(Enable)
  CANReceive3/3 -> Subsystem3/2(ID)
  CANReceive3/5 -> Terminator2/1

== system ultra/RX/288 290左后 ==
  CANReceive1 : ec5744lib/RapidECU_U4B/04CANCommunication/CANReceive  canmodule=0  canbuffer=44  canmessageid=hex2dec('288')  canmessagetype=Standard(11-bit ID)  datalength=8  sampletime=-1
      settings: SourceProductName=ECUCoder for MPC5744
  CANReceive2 : ec5744lib/RapidECU_U4B/04CANCommunication/CANReceive  canmodule=0  canbuffer=45  canmessageid=hex2dec('290')  canmessagetype=Standard(11-bit ID)  datalength=8  sampletime=-1
      settings: SourceProductName=ECUCoder for MPC5744
  MeaModule1 : ec5744lib/RapidECU_U4B/07Calibration/MeaModule  signal=CANOK_288
      settings: SourceProductName=ECUCoder for MPC5744
  MeaModule2 : ec5744lib/RapidECU_U4B/07Calibration/MeaModule  signal=CANOK_290
      settings: SourceProductName=ECUCoder for MPC5744
  Subsystem1 : Subsystem
  Subsystem2 : Subsystem
  Terminator1 : Terminator
  Terminator3 : Terminator
  wires:
  CANReceive1/5 -> Terminator3/1
  CANReceive1/2 -> MeaModule1/1
  CANReceive1/1 -> Subsystem2/Trigger
  CANReceive1/3 -> Subsystem2/2(ID)
  CANReceive1/4 -> Subsystem2/3(msg)
  MeaModule1/1 -> Subsystem2/1(Enable)
  CANReceive2/3 -> Subsystem1/2(ID)
  CANReceive2/4 -> Subsystem1/3(msg)
  CANReceive2/5 -> Terminator1/1
  CANReceive2/1 -> Subsystem1/Trigger
  MeaModule2/1 -> Subsystem1/1(Enable)
  CANReceive2/2 -> MeaModule2/1

== system ultra/RX/ebs ==
  CANReceive1 : ec5744lib/RapidECU_U4B/04CANCommunication/CANReceive  canmodule=2  canbuffer=31  canmessageid=hex2dec('402')  canmessagetype=Standard(11-bit ID)  datalength=8  sampletime=-1
      settings: SourceProductName=ECUCoder for MPC5744
  MeaModule8 : ec5744lib/RapidECU_U4B/07Calibration/MeaModule  signal=CANOK_402
      settings: SourceProductName=ECUCoder for MPC5744
  Subsystem3 : Subsystem
  Terminator3 : Terminator
  wires:
  CANReceive1/1 -> Subsystem3/Trigger
  CANReceive1/5 -> Terminator3/1
  MeaModule8/1 -> Subsystem3/1(Enable)
  CANReceive1/3 -> Subsystem3/2(ID)
  CANReceive1/4 -> Subsystem3/3(msg)
  CANReceive1/2 -> MeaModule8/1

== system ultra/RX/lcu——receive ==
  CANReceive : ec5744lib/RapidECU_U4B/04CANCommunication/CANReceive  canmodule=2  canbuffer=22  canmessageid=hex2dec('156')  canmessagetype=Standard(11-bit ID)  datalength=8  sampletime=-1
      settings: SourceProductName=ECUCoder for MPC5744
  Data Store Write : DataStoreWrite  DataStoreName=lcu_enable_185
  Data Store Write1 : DataStoreWrite  DataStoreName=lcu_enable_188
  Data Store Write2 : DataStoreWrite  DataStoreName=lcu_enable_185_1
  Data Store Write3 : DataStoreWrite  DataStoreName=lcu_enable_188_1
  Data Store Write4 : DataStoreWrite  DataStoreName=lcu_enable_184
  Data Store Write5 : DataStoreWrite  DataStoreName=lcu_enable_184_1
  Data Store Write6 : DataStoreWrite  DataStoreName=lcu_enable_189_1
  Data Store Write7 : DataStoreWrite  DataStoreName=lcu_enable_189
  Data Store Write8 : DataStoreWrite  DataStoreName=lcu_canok
  MATLAB Function : MATLAB Function  TreatAsAtomicUnit=on
  MeaModule : ec5744lib/RapidECU_U4B/07Calibration/MeaModule  signal=enable_185
      settings: SourceProductName=ECUCoder for MPC5744
  MeaModule1 : ec5744lib/RapidECU_U4B/07Calibration/MeaModule  signal=enable_185_1
      settings: SourceProductName=ECUCoder for MPC5744
  MeaModule11 : ec5744lib/RapidECU_U4B/07Calibration/MeaModule  signal=CANok
      settings: SourceProductName=ECUCoder for MPC5744
  MeaModule2 : ec5744lib/RapidECU_U4B/07Calibration/MeaModule  signal=enable_188
      settings: SourceProductName=ECUCoder for MPC5744
  MeaModule3 : ec5744lib/RapidECU_U4B/07Calibration/MeaModule  signal=enable_188_1
      settings: SourceProductName=ECUCoder for MPC5744
  MeaModule4 : ec5744lib/RapidECU_U4B/07Calibration/MeaModule  signal=enable_184
      settings: SourceProductName=ECUCoder for MPC5744
  MeaModule5 : ec5744lib/RapidECU_U4B/07Calibration/MeaModule  signal=enable_184_1
      settings: SourceProductName=ECUCoder for MPC5744
  MeaModule6 : ec5744lib/RapidECU_U4B/07Calibration/MeaModule  signal=enable_189
      settings: SourceProductName=ECUCoder for MPC5744
  MeaModule7 : ec5744lib/RapidECU_U4B/07Calibration/MeaModule  signal=enable_189_1
      settings: SourceProductName=ECUCoder for MPC5744
  Subsystem1 : Subsystem
  Terminator1 : Terminator
  Terminator2 : Terminator
  wires:
  CANReceive/2 -> MeaModule11/1
  CANReceive/4 -> Subsystem1/3(msg)
  CANReceive/3 -> Subsystem1/2(ID)
  CANReceive/5 -> Terminator2/1
  CANReceive/1 -> Subsystem1/Trigger
  MeaModule11/1 -> Data Store Write8/1, Subsystem1/1(Enable)
  Subsystem1/1(Out1) -> Terminator1/1
  MATLAB Function/2(enable_185_1) -> MeaModule1/1
  MeaModule1/1 -> Data Store Write2/1
  MATLAB Function/3(enable_188) -> MeaModule2/1
  MeaModule2/1 -> Data Store Write1/1
  MeaModule/1 -> Data Store Write/1
  MATLAB Function/1(enable_185) -> MeaModule/1
  MeaModule3/1 -> Data Store Write3/1
  MATLAB Function/4(enable_188_1) -> MeaModule3/1
  MATLAB Function/5(enable_184) -> MeaModule4/1
  MeaModule4/1 -> Data Store Write4/1
  MATLAB Function/6(enable_184_1) -> MeaModule5/1
  MeaModule5/1 -> Data Store Write5/1
  MATLAB Function/7(enable_189) -> MeaModule6/1
  MeaModule6/1 -> Data Store Write7/1
  MATLAB Function/8(enable_189_1) -> MeaModule7/1
  MeaModule7/1 -> Data Store Write6/1
  Subsystem1/2(m) -> MATLAB Function/1(m)

== system ultra/RX/工作站 ==
  CANReceive1 : ec5744lib/RapidECU_U4B/04CANCommunication/CANReceive  canmodule=2  canbuffer=51  canmessageid=hex2dec('20')  canmessagetype=Standard(11-bit ID)  datalength=6  sampletime=-1
      settings: SourceProductName=ECUCoder for MPC5744
  CANReceive2 : ec5744lib/RapidECU_U4B/04CANCommunication/CANReceive  canmodule=2  canbuffer=7  canmessageid=hex2dec('21')  canmessagetype=Standard(11-bit ID)  datalength=8  sampletime=-1
      settings: SourceProductName=ECUCoder for MPC5744
  Constant : Constant
  Data Store Write : DataStoreWrite  DataStoreName=CANOK_20
  MeaModule1 : ec5744lib/RapidECU_U4B/07Calibration/MeaModule  signal=CANOK_21
      settings: SourceProductName=ECUCoder for MPC5744
  MeaModule3 : ec5744lib/RapidECU_U4B/07Calibration/MeaModule  signal=CANOK_20
      settings: SourceProductName=ECUCoder for MPC5744
  Subsystem1 : Subsystem
  Subsystem3 : Subsystem
  Terminator1 : Terminator
  Terminator2 : Terminator
  wires:
  CANReceive1/4 -> Subsystem3/3(msg)
  CANReceive1/5 -> Terminator2/1
  CANReceive1/3 -> Subsystem3/2(ID)
  CANReceive1/1 -> Subsystem3/Trigger
  CANReceive1/2 -> Data Store Write/1, MeaModule3/1
  CANReceive2/3 -> Subsystem1/2(ID)
  CANReceive2/1 -> Subsystem1/Trigger
  MeaModule1/1 -> Subsystem1/1(Enable)
  CANReceive2/4 -> Subsystem1/3(msg)
  CANReceive2/5 -> Terminator1/1
  CANReceive2/2 -> MeaModule1/1
  Constant/1 -> Subsystem3/1(Enable)

== system ultra/RX/惯导 ==
  CANReceive1 : ec5744lib/RapidECU_U4B/04CANCommunication/CANReceive  canmodule=1  canbuffer=50  canmessageid=hex2dec('505')  canmessagetype=Standard(11-bit ID)  datalength=7  sampletime=-1
      settings: SourceProductName=ECUCoder for MPC5744
  CANReceive2 : ec5744lib/RapidECU_U4B/04CANCommunication/CANReceive  canmodule=1  canbuffer=49  canmessageid=hex2dec('502')  canmessagetype=Standard(11-bit ID)  datalength=7  sampletime=-1
      settings: SourceProductName=ECUCoder for MPC5744
  MeaModule1 : ec5744lib/RapidECU_U4B/07Calibration/MeaModule  signal=CANOK_500
      settings: SourceProductName=ECUCoder for MPC5744
  MeaModule2 : ec5744lib/RapidECU_U4B/07Calibration/MeaModule  signal=CANOK_502
      settings: SourceProductName=ECUCoder for MPC5744
  MeaModule3 : ec5744lib/RapidECU_U4B/07Calibration/MeaModule  signal=CANOK_505
      settings: SourceProductName=ECUCoder for MPC5744
  Subsystem1 : Subsystem
  Subsystem2 : Subsystem
  Subsystem3 : Subsystem
  Terminator1 : Terminator
  Terminator2 : Terminator
  Terminator3 : Terminator
  加速度 : ec5744lib/RapidECU_U4B/04CANCommunication/CANReceive  canmodule=1  canbuffer=48  canmessageid=hex2dec('500')  canmessagetype=Standard(11-bit ID)  datalength=7  sampletime=-1
      settings: SourceProductName=ECUCoder for MPC5744
  wires:
  加速度/5 -> Terminator3/1
  加速度/2 -> MeaModule1/1
  加速度/1 -> Subsystem2/Trigger
  加速度/3 -> Subsystem2/2(ID)
  加速度/4 -> Subsystem2/3(msg)
  MeaModule1/1 -> Subsystem2/1(Enable)
  CANReceive2/3 -> Subsystem1/2(ID)
  CANReceive2/4 -> Subsystem1/3(msg)
  CANReceive2/5 -> Terminator1/1
  CANReceive2/1 -> Subsystem1/Trigger
  MeaModule2/1 -> Subsystem1/1(Enable)
  CANReceive2/2 -> MeaModule2/1
  MeaModule3/1 -> Subsystem3/1(Enable)
  CANReceive1/4 -> Subsystem3/3(msg)
  CANReceive1/2 -> MeaModule3/1
  CANReceive1/5 -> Terminator2/1
  CANReceive1/3 -> Subsystem3/2(ID)
  CANReceive1/1 -> Subsystem3/Trigger

== system ultra/RX/转向——receive1 ==
  CANReceive1 : ec5744lib/RapidECU_U4B/04CANCommunication/CANReceive  canmodule=2  canbuffer=52  canmessageid=hex2dec('481')  canmessagetype=Standard(11-bit ID)  datalength=6  sampletime=-1
      settings: SourceProductName=ECUCoder for MPC5744
  CANReceive2 : ec5744lib/RapidECU_U4B/04CANCommunication/CANReceive  canmodule=2  canbuffer=53  canmessageid=hex2dec('81')  canmessagetype=Standard(11-bit ID)  datalength=1  sampletime=-1
      settings: SourceProductName=ECUCoder for MPC5744
  Data Store Write : DataStoreWrite  DataStoreName=zhuanxiangbaocuo
  MeaModule1 : ec5744lib/RapidECU_U4B/07Calibration/MeaModule  signal=CANOK_81
      settings: SourceProductName=ECUCoder for MPC5744
  MeaModule8 : ec5744lib/RapidECU_U4B/07Calibration/MeaModule  signal=CANOK_481
      settings: SourceProductName=ECUCoder for MPC5744
  Subsystem1 : Subsystem
  Subsystem3 : Subsystem
  Terminator1 : Terminator
  Terminator3 : Terminator
  wires:
  CANReceive1/1 -> Subsystem3/Trigger
  CANReceive1/4 -> Subsystem3/3(msg)
  CANReceive1/2 -> MeaModule8/1
  CANReceive1/5 -> Terminator3/1
  MeaModule8/1 -> Subsystem3/1(Enable)
  CANReceive1/3 -> Subsystem3/2(ID)
  MeaModule1/1 -> Data Store Write/1, Subsystem1/1(Enable)
  CANReceive2/3 -> Subsystem1/2(ID)
  CANReceive2/2 -> MeaModule1/1
  CANReceive2/4 -> Subsystem1/3(msg)
  CANReceive2/1 -> Subsystem1/Trigger
  CANReceive2/5 -> Terminator1/1
